simulink model "PreLQRSim"  (R2019b)
settings: Solver=VariableStepAuto  StartTime=0.0  StopTime=25  RelTol=1e-3
values from neighbouring files (symbols this model uses):
  CD_f = 0.6    [LQRcalc.m]    (also in LQRsetupvars.mat)
  CDa = 0.5    [LQRcalc.m]    (also in LQRsetupvars.mat)
  CL_f = 1.2    [LQRcalc.m]    (also in LQRsetupvars.mat)
  D = 0.1524    [LQRcalc.m]    (also in LQRsetupvars.mat)
  g = 9.81    [LQRcalc.m]    (also in LQRsetupvars.mat)
  hd = 3300    [LQRcalc.m]    (also in LQRsetupvars.mat)
  I = 0.1552    [LQRcalc.m]    (also in LQRsetupvars.mat)
  K = [-0.499999684437  6.32455931193  -4.18368770338; -0.500000315563  -6.32455132874  -4.18333456201]    [LQRsetupvars.mat]
  lmax = 0.0508    [LQRcalc.m]    (also in LQRsetupvars.mat)
  m = 45.06    [LQRcalc.m]    (also in LQRsetupvars.mat)
  rho = 1.225    [LQRcalc.m]    (also in LQRsetupvars.mat)
  servodelay = 0.08    [LQRcalc.m]    (also in LQRsetupvars.mat)
  Srefa = pi*D^2/4    (= 0.0182414692475)    [LQRcalc.m]    (also in LQRsetupvars.mat)
  vi = 279    [LQRcalc.m]    (also in LQRsetupvars.mat)
  w = 0.0508    [LQRcalc.m]    (also in LQRsetupvars.mat)
libraries: simulink x1
settings Model: OrderedModelArguments=off  Creator=anshu  LastModifiedBy=anshu

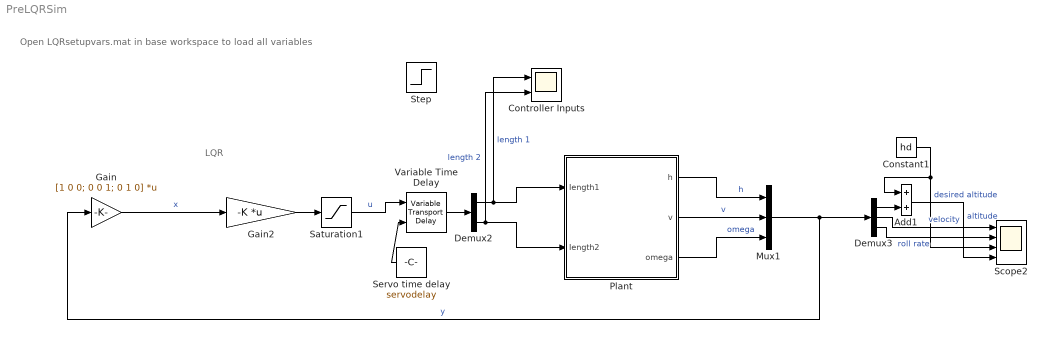
== system PreLQRSim ==
  note: Open LQRsetupvars.mat in base workspace to load all variables
  note: LQR
  Add1 : Sum
  Constant1 : Constant  Value=hd
  Controller Inputs : Scope  NumInputPorts=2
  Demux2 : Demux  Outputs=2
  Demux3 : Demux  Outputs=3
  Gain : Gain  Gain=[1 0 0; 0 0 1; 0 1 0]  Multiplication=Matrix(K*u)
  Gain2 : Gain  Gain=-K  Multiplication=Matrix(K*u) (u vector)
  Mux1 : Mux  Inputs=3
  Plant : Subsystem
  Saturation1 : Saturate  UpperLimit=lmax  LowerLimit=0
  Scope2 : Scope  NumInputPorts=4
  Servo time delay : Constant  Value=servodelay
  Step : Step  Time=5  Before=[0;0]  After=[lmax;lmax]  SampleTime=0
  Variable Time Delay : VariableTransportDelay  MaximumDelay=10
  wires:
  Demux3/1 -> Add1/2
  Mux1/1 -> Gain/1, Demux3/1  "y"
  Plant/2(v) -> Mux1/2  "v"
  Plant/1(h) -> Mux1/1  "h"
  Demux2/2 -> Plant/2(Iength2), Controller Inputs/2  "length 2"
  Constant1/1 -> Add1/1, Scope2/3  "desired altitude"
  Demux2/1 -> Controller Inputs/1, Plant/1(Iength1)  "length 1"
  Gain2/1 -> Saturation1/1
  Plant/3(omega) -> Mux1/3  "omega"
  Gain/1 -> Gain2/1  "x"
  Saturation1/1 -> Variable Time Delay/1  "u"
  Servo time delay/1 -> Variable Time Delay/2
  Add1/1 -> Scope2/4  "altitude"
  Demux3/2 -> Scope2/1  "velocity"
  Demux3/3 -> Scope2/2  "roll rate"
  Variable Time Delay/1 -> Demux2/1

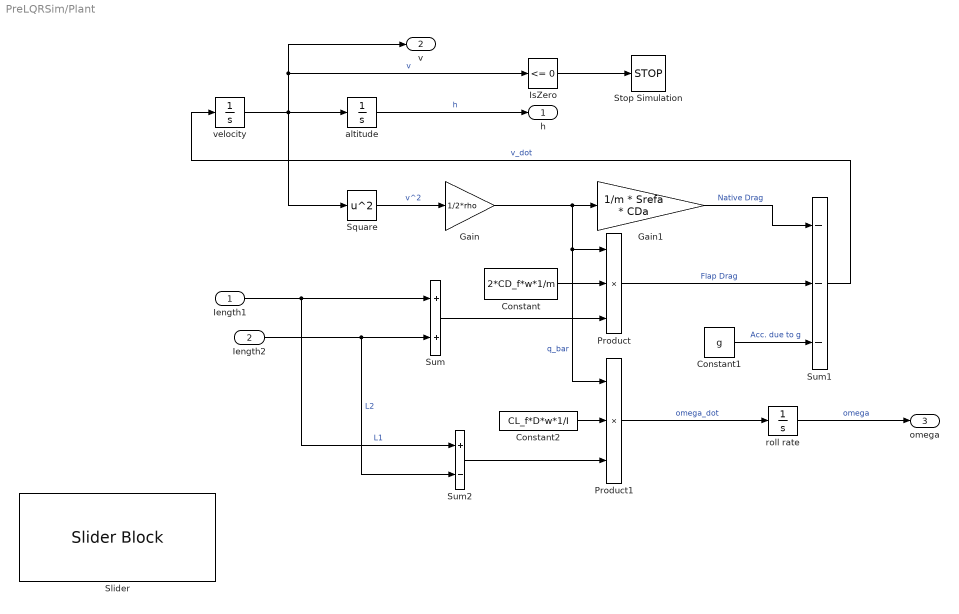
== system PreLQRSim/Plant ==
  Iength1 : Inport
  Iength2 : Inport  Port=2
  Constant : Constant  Value=2*CD_f*w*1/m
  Constant1 : Constant  Value=g
  Constant2 : Constant  Value=CL_f*D*w*1/I
  Gain : Gain  Gain=1/2*rho
  Gain1 : Gain  Gain=1/m * Srefa * CDa
  IsZero : simulink/Logic and Bit Operations/Compare To Zero  relop=<=  OutDataTypeStr=boolean
  Product : Product  Inputs=3
  Product1 : Product  Inputs=3
  Slider : SliderBlock
  Square : Math  Operator=square  SignedPower=off  SaturateOnIntegerOverflow=on
  Stop Simulation : Stop
  Sum : Sum  Inputs=2
  Sum1 : Sum  Inputs=---
  Sum2 : Sum  Inputs=+-
  altitude : Integrator  InitialCondition=hi - hd
  roll rate : Integrator  InitialCondition=4.737215909090909
  velocity : Integrator  InitialCondition=vi
  h : Outport
  v : Outport  Port=2
  omega : Outport  Port=3
  wires:
  Constant2/1 -> Product1/2
  Gain/1 -> Product1/1, Product/1, Gain1/1  "q_bar"
  Constant1/1 -> Sum1/3  "Acc. due to g"
  velocity/1 -> v/1, IsZero/1, altitude/1, Square/1  "v"
  altitude/1 -> h/1  "h"
  Gain1/1 -> Sum1/1  "Native Drag"
  Sum/1 -> Product/3
  Iength2/1 -> Sum2/2, Sum/2  "L2"
  Square/1 -> Gain/1  "v^2"
  Constant/1 -> Product/2
  Iength1/1 -> Sum2/1, Sum/1  "L1"
  Product/1 -> Sum1/2  "Flap Drag"
  Sum1/1 -> velocity/1  "v_dot"
  Product1/1 -> roll rate/1  "omega_dot"
  Sum2/1 -> Product1/3
  roll rate/1 -> omega/1  "omega"
  IsZero/1 -> Stop Simulation/1
